simulink model "sun_vector_test"  (R2016b)
settings: Solver=VariableStepAuto  StartTime=0.0  StopTime=1  RelTol=1e-3
values from neighbouring files (symbols this model uses):
  fsw_params = init_fsw_params()    [sun_vector_test_init.m]
libraries: GPS_time_lib x1, sgp4_lib_fsw x1, sun_vector_lib x1, time_coord_rotation_lib x1
settings Model: Creator=Taylor  LastModifiedBy=bijan

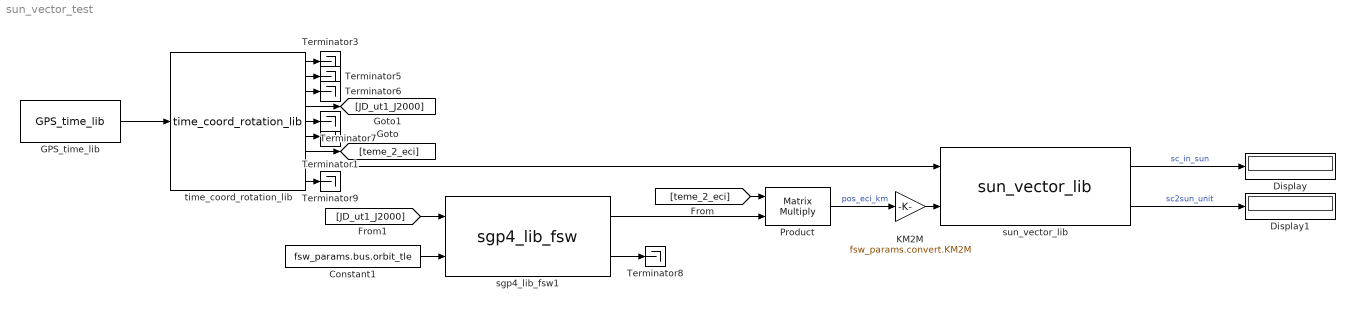
== system sun_vector_test ==
  Constant1 : Constant  Value=fsw_params.bus.orbit_tle
  Display : Display
  Display1 : Display
  GPS_time_lib : GPS_time_lib/GPS_time_lib
  KM2M : Gain  Gain=fsw_params.convert.KM2M
  Product : Product  Multiplication=Matrix(*)
  Terminator{1,3,5..9} (7 alike) : Terminator
  sgp4_lib_fsw1 : sgp4_lib_fsw/sgp4_lib_fsw
  sun_vector_lib : sun_vector_lib/sun_vector_lib
  time_coord_rotation_lib : time_coord_rotation_lib/time_coord_rotation_lib
  wires:
  sun_vector_lib/1 -> Display/1  "sc_in_sun"
  sun_vector_lib/2 -> Display1/1  "sc2sun_unit"
  Product/1 -> KM2M/1  "pos_eci_km"
  sgp4_lib_fsw1/2 -> Terminator8/1
  time_coord_rotation_lib/8 -> sun_vector_lib/1
  Constant1/1 -> sgp4_lib_fsw1/2
  KM2M/1 -> sun_vector_lib/2
  GPS_time_lib/1 -> time_coord_rotation_lib/1
  time_coord_rotation_lib/1 -> Terminator3/1
  time_coord_rotation_lib/2 -> Terminator5/1
  time_coord_rotation_lib/5 -> Terminator7/1
  time_coord_rotation_lib/7 -> [teme_2_eci]
  [teme_2_eci] -> Product/1
  time_coord_rotation_lib/4 -> [JD_ut1_J2000]
  [JD_ut1_J2000] -> sgp4_lib_fsw1/1
  sgp4_lib_fsw1/1 -> Product/2
  time_coord_rotation_lib/9 -> Terminator9/1
  time_coord_rotation_lib/6 -> Terminator1/1
  time_coord_rotation_lib/3 -> Terminator6/1
